simulink subsystem "Pupil_Diameter_Model_BaseLine"  (R2020a)
settings: Solver=VariableStepAuto  StartTime=0.0  StopTime=10.0  RelTol=1e-3
libraries: dspstat3 x1
settings Model: Creator=LAB-OREN3  LastModifiedBy=LAB-OREN3

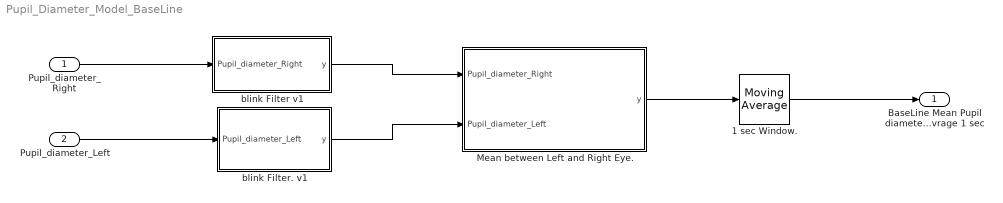
== system Pupil_Diameter_Model_BaseLine ==
  Pupil_diameter_Right : Inport
  Pupil_diameter_Left : Inport  Port=2
  1 sec Window. : dspstat3/Moving Average  Method=Sliding window  ForgettingFactorPort=off  SpecifyWindowLength=on  WindowLength=512  ForgettingFactor=0.9  SimulateUsing=Code generation
  Mean between Left and Right Eye. : MATLAB Function  TreatAsAtomicUnit=on
  blink Filter v1 : MATLAB Function  TreatAsAtomicUnit=on
  blink Filter. v1 : MATLAB Function  TreatAsAtomicUnit=on
  "BaseLine Mean Pupil diameter + Moving avrage 1 sec  " : Outport
  wires:
  Pupil_diameter_Right/1 -> blink Filter v1/1(Pupil_diameter_Right)
  blink Filter v1/1(y) -> Mean between Left and Right Eye./1(Pupil_diameter_Right)
  Pupil_diameter_Left/1 -> blink Filter. v1/1(Pupil_diameter_Left)
  blink Filter. v1/1(y) -> Mean between Left and Right Eye./2(Pupil_diameter_Left)
  1 sec Window./1 -> "BaseLine Mean Pupil diameter + Moving avrage 1 sec  "/1
  Mean between Left and Right Eye./1(y) -> 1 sec Window./1

== matlab function Pupil_Diameter_Model_BaseLine/blink Filter v1 ==
  data: Pupil_diameter_Right input; y output
function y = fcn(Pupil_diameter_Right)
    
  if Pupil_diameter_Right < 2.5 
      y = 2.5;
  elseif Pupil_diameter_Right > 8.0
      y = 8.0;
  else
      y = Pupil_diameter_Right;
  end
end

== matlab function Pupil_Diameter_Model_BaseLine/blink Filter. v1 ==
  data: Pupil_diameter_Left input; y output
function y = fcn(Pupil_diameter_Left)
    
  if Pupil_diameter_Left < 2.5 
      y = 2.5;
  elseif Pupil_diameter_Left > 8.0
      y = 8.0;
  else
      y = Pupil_diameter_Left;
  end
end

== matlab function Pupil_Diameter_Model_BaseLine/Mean between Left and Right Eye. ==
  data: Pupil_diameter_Right input; y output; Pupil_diameter_Left input
function y = fcn(Pupil_diameter_Right, Pupil_diameter_Left)
 
    
y = (Pupil_diameter_Right + Pupil_diameter_Left)/2;
